simulink model "Working_Voltage_Cutoff"  (R2024b)
settings: Solver=VariableStepAuto  StartTime=0.0  StopTime=3600  MaxStep=1  RelTol=1e-3
undefined symbols (not defined in the file): Ion, Lithium
libraries: spsBatteryLib x1, spsControlledCurrentSourceLib x1, spsVoltageMeasurementLib x1, spspowerguiLib x1
settings Model: Creator=balaj  LastModifiedBy=balaj

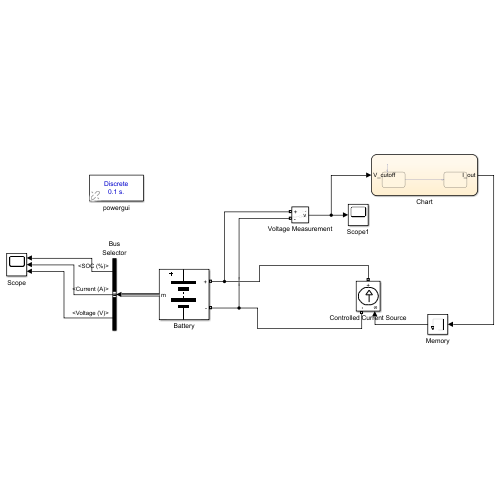
[thumbnail: Simulink's stored preview of the top-level diagram]
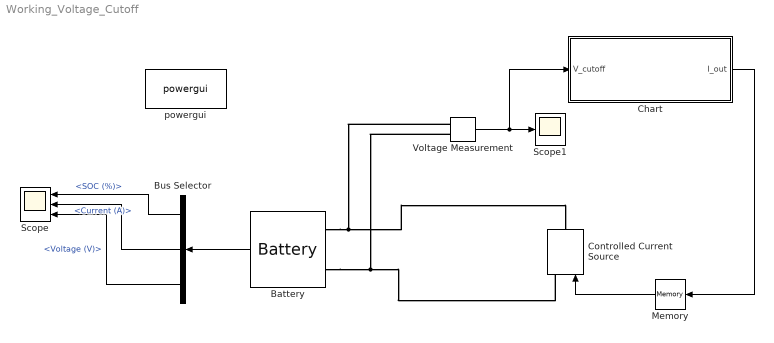
== system Working_Voltage_Cutoff ==
  Battery : spsBatteryLib/Battery  BatType=Lithium-Ion  NomV=3.7  NomQ=2.5  SOC=100  Batt_Tr=30  PresetModel=on  MaxQ=2.5  MinV=2.775  FullV=4.3068  Dis_rate=1.087  R=0.0148  Normal_OP=2.2609  expZone="[3.9974     0.12283]"
  Bus Selector : BusSelector  OutputSignals=SOC (%),Current (A),Voltage (V)
  Chart : Stateflow chart  TreatAsAtomicUnit=on
  Controlled Current Source : spsControlledCurrentSourceLib/Controlled Current Source  Initialize=on  Source_Type=AC  Amplitude=0  Phase=0  Frequency=0  Measurements=Current
  Memory : Memory  InitialCondition=-2.5
  Scope : Scope  NumInputPorts=3
  Scope1 : Scope
  Voltage Measurement : spsVoltageMeasurementLib/Voltage Measurement  PhasorSimulation=off  OutputType=Complex  PSBequivalent=0
  powergui : spspowerguiLib/powergui  Priority=1  SimulationMode=Discrete  SampleTime=0.1  frequency=60  Iterations=50  frequencyindice=0  Pbase=100e6  ErrMax=1e-4  UnitsV=kV  UnitsW=MW  buscounter=0  FunctionMessages=off  echomessages=off  EnableUseOfTLC=off  CurrentSourceSwitches=off  DisableSnubberDevices=off  DisableRonSwitches=off  DisableVfSwitches=off  DisplayEquations=off  AutomaticDiscreteSolvers=off  SolverType=Tustin/Backward Euler (TBE)  Interpol=off  ExternalGateDelay=off  methode=off  Ts=100  x0status=blocks  SPID=on  SwTol=0  HookPort=off  NonlinearTolerance=1e-4  nMaxIteration=100  ContinueOnMaxIteration=off  RestoreLinks=warning  ResistiveCurrentMeasurement=off  Frange=[0:2:500]  Ylog=off  Xlog=on  ShowGrid=off  save=off  variable=ZData  structure=0  ZoomFFT=off  StartTime=0.0  cycles=1  DisplayStyle=1  fundamental=60  FreqAxis=off  MaxFrequency=1000  frequencyindicesteady=1  RmsSteady=1  display=off
  wires:
  Battery/1 -> Bus Selector/1
  Bus Selector/1 -> Scope/1  "<SOC (%)>"
  Bus Selector/2 -> Scope/2  "<Current (A)>"
  Bus Selector/3 -> Scope/3  "<Voltage (V)>"
  Voltage Measurement/1 -> Chart/1(V_cutoff), Scope1/1
  Chart/1(I_out) -> Memory/1
  Memory/1 -> Controlled Current Source/1
  connections:
  Battery/LConn1 -- Voltage Measurement/LConn1 -- Controlled Current Source/RConn1
  Battery/LConn2 -- Voltage Measurement/LConn2 -- Controlled Current Source/LConn1

== stateflow chart Working_Voltage_Cutoff/Chart ==
  state StateA
    entry:
    I_out=-2.5
  state StateB
    entry:
    I_out=0
  (default) -> StateA
  StateA -> StateB : [V_cutoff<=2.5]
  data: V_cutoff input; I_out output
